simulink model "sine_test"  (R2021a)
settings: Solver=VariableStepAuto  StartTime=0.0  StopTime=1024  RelTol=1e-3
libraries: xbsIndex_r4 x17
settings Model: Creator=rfsoc-dev  LastModifiedBy=rfsoc-dev

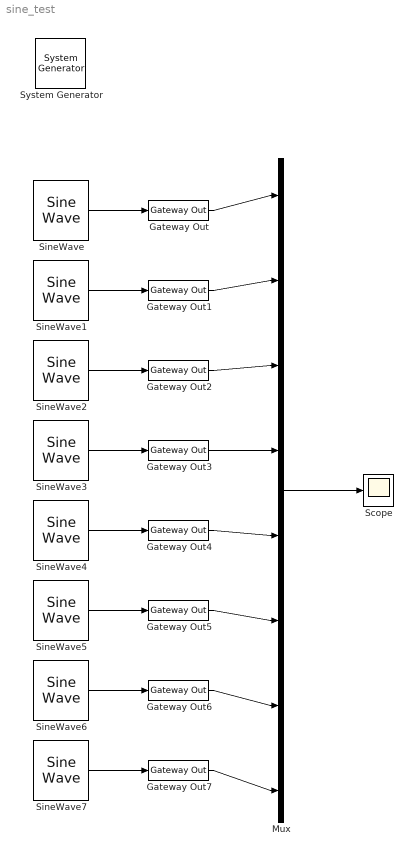
== system sine_test ==
  " System Generator" : xbsIndex_r4/ System Generator  Tag=genX  xilinxfamily=kintex7  part=xc7k325t  speed=-3  package=fbg676  synthesis_tool=Vivado  clock_wrapper=Clock Enables  directory=./netlist  proj_type=Vivado  Synth_file=Vivado Synthesis Defaults  Impl_file=Vivado Implementation Defaults  testbench=off  simulink_period=1  sysclk_period=10  dcm_input_clock_period=10  incr_netlist=off  trim_vbits=Everywhere in SubSystem  dbl_ovrd=According to Block Masks  core_generation=According to Block Masks  run_coregen=off  deprecated_control=off  eval_field=0  block_type=sysgen
  Gateway Out{,1..7} (8 alike) : xbsIndex_r4/Gateway Out  inherit_from_input=off  hdl_port=on  rows=1  columns=1  UseAsDAC=off  DACChannel='1'  interface=None  automatic_assignment=on  address_offset=hex2dec('00')  intf_name=''  intf_description=''  timing_constraint=None  locs_specified=off  LOCs={}  io_standard={}  block_type=gatewayout
  Mux : Mux  Inputs=8
  Scope : Scope
  SineWave : xbsIndex_r4/Sine Wave  Input_format=Frequency  output_frequency=1/512  phase_offset_angles=0  output_selection=Sine  sfdr=95  explicit_period=on  period=1  simulation_type=fast_sim  simulation_model=sysgen:dds_macro  block_type=dds_macro
  SineWave1 : xbsIndex_r4/Sine Wave  Input_format=Frequency  output_frequency=1/512  phase_offset_angles=1/4096  output_selection=Sine  sfdr=95  explicit_period=on  period=1  simulation_type=fast_sim  simulation_model=sysgen:dds_macro  block_type=dds_macro
  SineWave2 : xbsIndex_r4/Sine Wave  Input_format=Frequency  output_frequency=1/512  phase_offset_angles=2/4096  output_selection=Sine  sfdr=95  explicit_period=on  period=1  simulation_type=fast_sim  simulation_model=sysgen:dds_macro  block_type=dds_macro
  SineWave3 : xbsIndex_r4/Sine Wave  Input_format=Frequency  output_frequency=1/512  phase_offset_angles=3/4096  output_selection=Sine  sfdr=95  explicit_period=on  period=1  simulation_type=fast_sim  simulation_model=sysgen:dds_macro  block_type=dds_macro
  SineWave4 : xbsIndex_r4/Sine Wave  Input_format=Frequency  output_frequency=1/512  phase_offset_angles=4/4096  output_selection=Sine  sfdr=95  explicit_period=on  period=1  simulation_type=fast_sim  simulation_model=sysgen:dds_macro  block_type=dds_macro
  SineWave5 : xbsIndex_r4/Sine Wave  Input_format=Frequency  output_frequency=1/512  phase_offset_angles=5/4096  output_selection=Sine  sfdr=95  explicit_period=on  period=1  simulation_type=fast_sim  simulation_model=sysgen:dds_macro  block_type=dds_macro
  SineWave6 : xbsIndex_r4/Sine Wave  Input_format=Frequency  output_frequency=1/512  phase_offset_angles=6/4096  output_selection=Sine  sfdr=95  explicit_period=on  period=1  simulation_type=fast_sim  simulation_model=sysgen:dds_macro  block_type=dds_macro
  SineWave7 : xbsIndex_r4/Sine Wave  Input_format=Frequency  output_frequency=1/512  phase_offset_angles=7/4096  output_selection=Sine  sfdr=95  explicit_period=on  period=1  simulation_type=fast_sim  simulation_model=sysgen:dds_macro  block_type=dds_macro
  wires:
  SineWave/1 -> Gateway Out/1
  SineWave1/1 -> Gateway Out1/1
  SineWave3/1 -> Gateway Out3/1
  SineWave2/1 -> Gateway Out2/1
  Mux/1 -> Scope/1
  SineWave6/1 -> Gateway Out6/1
  SineWave7/1 -> Gateway Out7/1
  SineWave5/1 -> Gateway Out5/1
  SineWave4/1 -> Gateway Out4/1
  Gateway Out/1 -> Mux/1
  Gateway Out1/1 -> Mux/2
  Gateway Out2/1 -> Mux/3
  Gateway Out3/1 -> Mux/4
  Gateway Out4/1 -> Mux/5
  Gateway Out5/1 -> Mux/6
  Gateway Out6/1 -> Mux/7
  Gateway Out7/1 -> Mux/8
